simulink model "Exercitiul5"  (R2016a)
settings: Solver=VariableStepDiscrete  StartTime=0.0  StopTime=28800  RelTol=1e-3
undefined symbols (not defined in the file): m, n
settings Model: Creator=Cristina  LastModifiedBy=Cristina

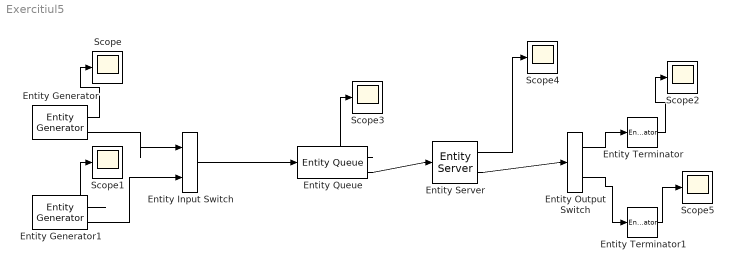
== system Exercitiul5 ==
  Entity Input Switch : EntityInputSwitch  InputPortMessageModes=m,m  OutputPortMessageModes=m
  Entity Output Switch : EntityOutputSwitch  InputPortMessageModes=m  OutputPortMessageModes=m,m  SwitchingCriterion=From attribute  SwitchAttributeName=Attribute1
  Entity Generator : EntityGenerator  OutputPortMessageModes=n,m  TimeSource=MATLAB action  IntergenerationTimeAction=dt = 60 + 720 * rand;  NumberEntitiesDeparted=on  EntityType=Structured  EntityTypeName=Entity  EntityPriority=30
      settings: OutputPortMap=o0,o3
  Entity Generator1 : EntityGenerator  OutputPortMessageModes=n,m  TimeSource=MATLAB action  IntergenerationTimeAction=dt = 70 + 130 * rand;  NumberEntitiesDeparted=on  EntityType=Structured  EntityTypeName=Entity  EntityPriority=30
      settings: OutputPortMap=o0,o3
  Entity Queue : EntityQueue  InputPortMessageModes=m  OutputPortMessageModes=n,m  Capacity=300  QueueType=Priority  PrioritySource=entitySys.priority  SortingDirection=Descending  AverageQueueLength=on
      settings: OutputPortMap=o3,o5
  Entity Server : EntityServer  InputPortMessageModes=m  OutputPortMessageModes=n,m  Capacity=1  EntryAction=|  NumberEntitiesDeparted=on
      | if (entitySys.priority == 20)
      |     dt = 210 + 180 * rand;
      | else
      |     dt = 70 + 130 * rand;
      | end
      settings: OutputPortMap=o0,o9
  Entity Terminator : EntityTerminator  InputPortMessageModes=m  NumberEntitiesArrived=on
      settings: OutputPortMap=o0
  Entity Terminator1 : EntityTerminator  InputPortMessageModes=m  NumberEntitiesArrived=on
      settings: OutputPortMap=o0
  Scope{,1..5} (6 alike) : Scope
  wires:
  Entity Generator/2 -> Entity Input Switch/1
  Entity Generator1/2 -> Entity Input Switch/2
  Entity Input Switch/1 -> Entity Queue/1
  Entity Queue/2 -> Entity Server/1
  Entity Server/2 -> Entity Output Switch/1
  Entity Generator/1 -> Scope/1
  Entity Generator1/1 -> Scope1/1
  Entity Queue/1 -> Scope3/1
  Entity Server/1 -> Scope4/1
  Entity Output Switch/1 -> Entity Terminator/1
  Entity Output Switch/2 -> Entity Terminator1/1
  Entity Terminator/1 -> Scope2/1
  Entity Terminator1/1 -> Scope5/1
